simulink model "mrefrobotarm_modified_previous_y_previous_u_previous_ref_pert"  (R2018b)
settings: Solver=FixedStepAuto  StartTime=0.0  StopTime=10  RelTol=1e-3  AbsTol=1e-6
undefined symbols (not defined in the file or in its folder): cc, options
libraries: neural x714, simulink x1
(part 18 of 26)

== system mrefrobotarm_modified_previous_y_previous_u_previous_ref_pert/sd=0.01/Layer 3/Delays 1 ==
  "p{3}" : Inport  PortDimensions=30
      mask Display: e = 0.06;c1 = [120 230 180]/255;c2 = ([120 230 180]+0)/(256+128);c3 = ([120 230 180]+128)/(256+128);patch([0 1 1 0],[0 0 1 1],c1);patch([0 1 1 1-e 1-e 0+e],[0 0 1 1-e 0+e 0+e],c2);patch([0 0 1 1-e 0+e 0+e],[0 1 1 1-e 1-e 0+e],c3);plot([0 1 1 0 0],[0 0 1 1 0]);
  mux : Mux  Inputs=1
      mask Display: e = 0.06;c1 = [120 150 230]/255;c2 = ([120 150 230]+0)/383;c3 = ([120 150 230]+128)/383;patch([0 1 1 0],[0 0 1 1],c1);patch([0 1 1 1-e 1-e 0+e],[0 0 1 1-e 0+e 0+e],c2);patch([0 0 1 1-e 0+e 0+e],[0 1 1 1-e 1-e 0+e],c3);plot([0 1 1 0 0],[0 0 1 1 0]);disp('Mux')
  "pd{3,2}" : Outport
      mask Display: e = 0.06;c1 = [120 230 180]/255;c2 = ([120 230 180]+0)/(256+128);c3 = ([120 230 180]+128)/(256+128);patch([0 1 1 0],[0 0 1 1],c1);patch([0 1 1 1-e 1-e 0+e],[0 0 1 1-e 0+e 0+e],c2);patch([0 0 1 1-e 0+e 0+e],[0 1 1 1-e 1-e 0+e],c3);plot([0 1 1 0 0],[0 0 1 1 0]);
  wires:
  "p{3}"/1 -> mux/1
  mux/1 -> "pd{3,2}"/1

== system mrefrobotarm_modified_previous_y_previous_u_previous_ref_pert/sd=0.01/Layer 3/LW{3,2} ==
  "ad{3,2}" : Inport  PortDimensions=30
      mask Display: e = 0.06;c1 = [120 230 180]/255;c2 = ([120 230 180]+0)/(256+128);c3 = ([120 230 180]+128)/(256+128);patch([0 1 1 0],[0 0 1 1],c1);patch([0 1 1 1-e 1-e 0+e],[0 0 1 1-e 0+e 0+e],c2);patch([0 0 1 1-e 0+e 0+e],[0 1 1 1-e 1-e 0+e],c3);plot([0 1 1 0 0],[0 0 1 1 0]);
  "IW{3,2}(1,:)'" : Constant  Value=[-0.64661080882801724722952485535643063485622406005859375;0.122506844708924533815519453128217719495296478271484375;-0.1598857817103115086521114562856382690370082855224609375;0.763629292094280653913074274896644055843353271484375;0.64783885944440944282263217246509157121181488037109375;-0.36352935298451505286010387862916104495525360107421875;-0.43128711595355684327302014935412444174289703369140625;-0.5895897301103618648454585127183236181735992431640625;-0.08369026570109527884966382771381177008152008056640625;-0.1004753957202015046679122178829857148230075836181640625;-0.32808404490869491620941289511392824351787567138671875;0.32998136189090920833422160285408608615398406982421875;-0.4486208899527432958365125159616582095623016357421875;0.0261813632498970362549872703539222129620611667633056640625;0.282027752833665268372698164967005141079425811767578125;-0.018494292466418822684648404219842632301151752471923828125;-0.1400613205037356812088233937174663878977298736572265625;0.017723947989941535308133779835770837962627410888671875;-0.012245723361617721902661060084938071668148040771484375;0.10735791327470788070197471597566618584096431732177734375;-0.12221158004853945044931862184967030771076679229736328125;-0.101564950316621105397274504866800270974636077880859375;0.022351703842111880771170717707718722522258758544921875;-0.075846949807921060227045018109492957592010498046875;0.09973817654474255445240515882687759585678577423095703125;0.1126567720389630988808704614712041802704334259033203125;0.023371450347008236592127872199853300116956233978271484375;0.297336107042620145790579044842161238193511962890625;-0.319404206955927250088933533334056846797466278076171875;-0.48364044976087694482913548199576325714588165283203125]
      mask Display: e = 0.06;c1 = [120 150 230]/255;c2 = ([120 150 230]+0)/383;c3 = ([120 150 230]+128)/383;patch([0 1 1 0],[0 0 1 1],c1);patch([0 1 1 1-e 1-e 0+e],[0 0 1 1-e 0+e 0+e],c2);patch([0 0 1 1-e 0+e 0+e],[0 1 1 1-e 1-e 0+e],c3);plot([0 1 1 0 0],[0 0 1 1 0]);disp('weights');
  Mux : Mux  Inputs=1
      mask Display: e = 0.06;c1 = [120 150 230]/255;c2 = ([120 150 230]+0)/383;c3 = ([120 150 230]+128)/383;patch([0 1 1 0],[0 0 1 1],c1);patch([0 1 1 1-e 1-e 0+e],[0 0 1 1-e 0+e 0+e],c2);patch([0 0 1 1-e 0+e 0+e],[0 1 1 1-e 1-e 0+e],c3);plot([0 1 1 0 0],[0 0 1 1 0]);disp('Mux');
  dotprod1 : neural/Weight Functions/dotprod
  "lz{3,2}" : Outport
      mask Display: e = 0.06;c1 = [120 230 180]/255;c2 = ([120 230 180]+0)/(256+128);c3 = ([120 230 180]+128)/(256+128);patch([0 1 1 0],[0 0 1 1],c1);patch([0 1 1 1-e 1-e 0+e],[0 0 1 1-e 0+e 0+e],c2);patch([0 0 1 1-e 0+e 0+e],[0 1 1 1-e 1-e 0+e],c3);plot([0 1 1 0 0],[0 0 1 1 0]);
  wires:
  "IW{3,2}(1,:)'"/1 -> dotprod1/1
  "ad{3,2}"/1 -> dotprod1/2
  dotprod1/1 -> Mux/1
  Mux/1 -> "lz{3,2}"/1

== system mrefrobotarm_modified_previous_y_previous_u_previous_ref_pert/sd=0.1/Layer 1/Delays 1 ==
  "p{1}" : Inport  PortDimensions=10
      mask Display: e = 0.06;c1 = [120 230 180]/255;c2 = ([120 230 180]+0)/(256+128);c3 = ([120 230 180]+128)/(256+128);patch([0 1 1 0],[0 0 1 1],c1);patch([0 1 1 1-e 1-e 0+e],[0 0 1 1-e 0+e 0+e],c2);patch([0 0 1 1-e 0+e 0+e],[0 1 1 1-e 1-e 0+e],c3);plot([0 1 1 0 0],[0 0 1 1 0]);
  mux : Mux  Inputs=1
      mask Display: e = 0.06;c1 = [120 150 230]/255;c2 = ([120 150 230]+0)/383;c3 = ([120 150 230]+128)/383;patch([0 1 1 0],[0 0 1 1],c1);patch([0 1 1 1-e 1-e 0+e],[0 0 1 1-e 0+e 0+e],c2);patch([0 0 1 1-e 0+e 0+e],[0 1 1 1-e 1-e 0+e],c3);plot([0 1 1 0 0],[0 0 1 1 0]);disp('Mux')
  "pd{1,1}" : Outport
      mask Display: e = 0.06;c1 = [120 230 180]/255;c2 = ([120 230 180]+0)/(256+128);c3 = ([120 230 180]+128)/(256+128);patch([0 1 1 0],[0 0 1 1],c1);patch([0 1 1 1-e 1-e 0+e],[0 0 1 1-e 0+e 0+e],c2);patch([0 0 1 1-e 0+e 0+e],[0 1 1 1-e 1-e 0+e],c3);plot([0 1 1 0 0],[0 0 1 1 0]);
  wires:
  "p{1}"/1 -> mux/1
  mux/1 -> "pd{1,1}"/1

== system mrefrobotarm_modified_previous_y_previous_u_previous_ref_pert/sd=0.1/Layer 1/IW{1,1} ==
  "pd{1,1}" : Inport  PortDimensions=10
      mask Display: e = 0.06;c1 = [120 230 180]/255;c2 = ([120 230 180]+0)/(256+128);c3 = ([120 230 180]+128)/(256+128);patch([0 1 1 0],[0 0 1 1],c1);patch([0 1 1 1-e 1-e 0+e],[0 0 1 1-e 0+e 0+e],c2);patch([0 0 1 1-e 0+e 0+e],[0 1 1 1-e 1-e 0+e],c3);plot([0 1 1 0 0],[0 0 1 1 0]);
  "IW{1,1}(1,:)'" : Constant  Value=[5.6909541676817223532225398230366408824920654296875;-4.44478226511212515248416821123100817203521728515625;-0.69604359596750364769235375206335447728633880615234375;1.619034904975128252857530242181383073329925537109375;1.860125505340791907116226866492070257663726806640625;0.82729353143531325631698791767121292650699615478515625;-0.76269359990041951657957497445750050246715545654296875;-0.227256476361503645389205985338776372373104095458984375;0.461910119411805875078158578617149032652378082275390625;0.795152404857870198640057424199767410755157470703125]
      mask Display: e = 0.06;c1 = [120 150 230]/255;c2 = ([120 150 230]+0)/383;c3 = ([120 150 230]+128)/383;patch([0 1 1 0],[0 0 1 1],c1);patch([0 1 1 1-e 1-e 0+e],[0 0 1 1-e 0+e 0+e],c2);patch([0 0 1 1-e 0+e 0+e],[0 1 1 1-e 1-e 0+e],c3);plot([0 1 1 0 0],[0 0 1 1 0]);disp('Weights');
  "IW{1,1}(10,:)'" : Constant  Value=[3.77468306817619936310848061111755669116973876953125;-3.808687190450835924337980031850747764110565185546875;0.51746378608962484424438343921792693436145782470703125;-0.55078587150574531694502411482972092926502227783203125;-2.32173055805795680583969442523084580898284912109375;1.0626571361019880868070686119608581066131591796875;-0.23445984031463940056028150138445198535919189453125;-0.6493437208006149763406256170128472149372100830078125;1.4139047823904089540292261517606675624847412109375;0.617736660902912237958162222639657557010650634765625]
      mask Display: e = 0.06;c1 = [120 150 230]/255;c2 = ([120 150 230]+0)/383;c3 = ([120 150 230]+128)/383;patch([0 1 1 0],[0 0 1 1],c1);patch([0 1 1 1-e 1-e 0+e],[0 0 1 1-e 0+e 0+e],c2);patch([0 0 1 1-e 0+e 0+e],[0 1 1 1-e 1-e 0+e],c3);plot([0 1 1 0 0],[0 0 1 1 0]);disp('Weights');
  "IW{1,1}(11,:)'" : Constant  Value=[-0.1323443689410443990794874480343423783779144287109375;2.220754767172888222148685599677264690399169921875;11.4959613192428538042122454498894512653350830078125;-14.297590523719986066453202511183917522430419921875;-0.29115584099639824078309402466402389109134674072265625;3.022911440482079825642358628101646900177001953125;-0.112180835536244638550584795666509307920932769775390625;-0.981954934883976005011163579183630645275115966796875;0.10516967591617638888568109223342617042362689971923828125;1.8918544992947972094299302625586278736591339111328125]
      mask Display: e = 0.06;c1 = [120 150 230]/255;c2 = ([120 150 230]+0)/383;c3 = ([120 150 230]+128)/383;patch([0 1 1 0],[0 0 1 1],c1);patch([0 1 1 1-e 1-e 0+e],[0 0 1 1-e 0+e 0+e],c2);patch([0 0 1 1-e 0+e 0+e],[0 1 1 1-e 1-e 0+e],c3);plot([0 1 1 0 0],[0 0 1 1 0]);disp('Weights');
  "IW{1,1}(12,:)'" : Constant  Value=[0.72754685821430609138360523502342402935028076171875;-0.6570666137841676412989500022376887500286102294921875;-0.307371304859638871942451032737153582274913787841796875;-0.058820122292903016802956273068048176355659961700439453125;0.161741526428527071512775137307471595704555511474609375;-0.05792305025135065232877451535387081094086170196533203125;1.180419195584523794906317561981268227100372314453125;-0.51747520174959993344288022854016162455081939697265625;0.305574366681974851633896150815417058765888214111328125;0.2273021954544744149817603329211124219000339508056640625]
      mask Display: e = 0.06;c1 = [120 150 230]/255;c2 = ([120 150 230]+0)/383;c3 = ([120 150 230]+128)/383;patch([0 1 1 0],[0 0 1 1],c1);patch([0 1 1 1-e 1-e 0+e],[0 0 1 1-e 0+e 0+e],c2);patch([0 0 1 1-e 0+e 0+e],[0 1 1 1-e 1-e 0+e],c3);plot([0 1 1 0 0],[0 0 1 1 0]);disp('Weights');
  "IW{1,1}(13,:)'" : Constant  Value=[0.92475187713074102902055528829805552959442138671875;-0.7246700213142720503611826643464155495166778564453125;-0.54231701267272092170657060705707408487796783447265625;-0.74731381930544571456920266427914611995220184326171875;-0.37753760663786517515205787276499904692173004150390625;0.69288465345196315059439484684844501316547393798828125;-0.6787969769950346066167412573122419416904449462890625;1.4879723311172383670708541103522293269634246826171875;1.0728866219769777057280180088127963244915008544921875;-0.0257443446317741110596077902528122649528086185455322265625]
      mask Display: e = 0.06;c1 = [120 150 230]/255;c2 = ([120 150 230]+0)/383;c3 = ([120 150 230]+128)/383;patch([0 1 1 0],[0 0 1 1],c1);patch([0 1 1 1-e 1-e 0+e],[0 0 1 1-e 0+e 0+e],c2);patch([0 0 1 1-e 0+e 0+e],[0 1 1 1-e 1-e 0+e],c3);plot([0 1 1 0 0],[0 0 1 1 0]);disp('Weights');
  "IW{1,1}(14,:)'" : Constant  Value=[-0.39658704580621850777077952443505637347698211669921875;-2.570658577061915917028045441838912665843963623046875;2.097471663743316838690589065663516521453857421875;-0.182743645563124779140906639440800063312053680419921875;3.173197263880643159694727728492580354213714599609375;-2.566203225034959789496724624768830835819244384765625;0.28465571871831463202084933072910644114017486572265625;0.53816262288512628497727519061299972236156463623046875;1.148349370577057104725327008054591715335845947265625;-0.77361570994371497977937224277411587536334991455078125]
      mask Display: e = 0.06;c1 = [120 150 230]/255;c2 = ([120 150 230]+0)/383;c3 = ([120 150 230]+128)/383;patch([0 1 1 0],[0 0 1 1],c1);patch([0 1 1 1-e 1-e 0+e],[0 0 1 1-e 0+e 0+e],c2);patch([0 0 1 1-e 0+e 0+e],[0 1 1 1-e 1-e 0+e],c3);plot([0 1 1 0 0],[0 0 1 1 0]);disp('Weights');
  "IW{1,1}(15,:)'" : Constant  Value=[-1.233071996055086660959432265372015535831451416015625;3.729934935631209924622453399933874607086181640625;-0.69194072859403676911682623540400527417659759521484375;-0.06934859583439123564829742463189177215099334716796875;-1.3472043188516165113099987138411961495876312255859375;0.088223980720888273143742708271020092070102691650390625;-0.7180079381626434109620049639488570392131805419921875;-0.050715270149810497135600684259770787321031093597412109375;-0.79841827776868690147438201165641658008098602294921875;0.6403567898287889637032321843435056507587432861328125]
      mask Display: e = 0.06;c1 = [120 150 230]/255;c2 = ([120 150 230]+0)/383;c3 = ([120 150 230]+128)/383;patch([0 1 1 0],[0 0 1 1],c1);patch([0 1 1 1-e 1-e 0+e],[0 0 1 1-e 0+e 0+e],c2);patch([0 0 1 1-e 0+e 0+e],[0 1 1 1-e 1-e 0+e],c3);plot([0 1 1 0 0],[0 0 1 1 0]);disp('Weights');
  "IW{1,1}(16,:)'" : Constant  Value=[-0.4501147463957007044399460937711410224437713623046875;-0.4634484641641158919611598321353085339069366455078125;-1.074232972538778252413749214611016213893890380859375;2.414632291410705011713844214682467281818389892578125;1.5871822908788753014874828295432962477207183837890625;-0.936050277862158441877227232907898724079132080078125;-0.301929298988273753234778951082262210547924041748046875;0.2105845785872021147522303863297565840184688568115234375;-0.389900971878246072055418380841729231178760528564453125;-0.34803444346408973775197637223755009472370147705078125]
      mask Display: e = 0.06;c1 = [120 150 230]/255;c2 = ([120 150 230]+0)/383;c3 = ([120 150 230]+128)/383;patch([0 1 1 0],[0 0 1 1],c1);patch([0 1 1 1-e 1-e 0+e],[0 0 1 1-e 0+e 0+e],c2);patch([0 0 1 1-e 0+e 0+e],[0 1 1 1-e 1-e 0+e],c3);plot([0 1 1 0 0],[0 0 1 1 0]);disp('Weights');
  "IW{1,1}(17,:)'" : Constant  Value=[-0.99686635965547853999169092276133596897125244140625;-4.42672798675833245596322740311734378337860107421875;0.52979427551061120116315805717022158205509185791015625;6.21254233611867245912208090885542333126068115234375;0.5363341023376178018366999822319485247135162353515625;-1.0699517545959584818859866572893224656581878662109375;2.39944942593691745713613272528164088726043701171875;0.260939315381722158893040841576294042170047760009765625;0.2099266373906171490038019555868231691420078277587890625;-0.994914330157364634743544229422695934772491455078125]
      mask Display: e = 0.06;c1 = [120 150 230]/255;c2 = ([120 150 230]+0)/383;c3 = ([120 150 230]+128)/383;patch([0 1 1 0],[0 0 1 1],c1);patch([0 1 1 1-e 1-e 0+e],[0 0 1 1-e 0+e 0+e],c2);patch([0 0 1 1-e 0+e 0+e],[0 1 1 1-e 1-e 0+e],c3);plot([0 1 1 0 0],[0 0 1 1 0]);disp('Weights');
  "IW{1,1}(18,:)'" : Constant  Value=[-0.821393751051058274015304050408303737640380859375;-0.01417692834606891494342306714315782301127910614013671875;2.038276852058502175424337110598571598529815673828125;-2.792063261322187628366009448654949665069580078125;0.2963152941576634447073956835083663463592529296875;1.2640438926848338585529063493595458567142486572265625;-0.435348179999016704488923323879134841263294219970703125;-0.73195572965866928516476264121592976152896881103515625;0.452296877126517726797061413890332914888858795166015625;0.4165847639021185155883131301379762589931488037109375]
      mask Display: e = 0.06;c1 = [120 150 230]/255;c2 = ([120 150 230]+0)/383;c3 = ([120 150 230]+128)/383;patch([0 1 1 0],[0 0 1 1],c1);patch([0 1 1 1-e 1-e 0+e],[0 0 1 1-e 0+e 0+e],c2);patch([0 0 1 1-e 0+e 0+e],[0 1 1 1-e 1-e 0+e],c3);plot([0 1 1 0 0],[0 0 1 1 0]);disp('Weights');
  "IW{1,1}(19,:)'" : Constant  Value=[-0.021101967185585483732790379463040153495967388153076171875;1.04526769321619639185882988385856151580810546875;1.5178135598712625409234533435665071010589599609375;-3.477264311782526373661994512076489627361297607421875;-0.65282281292846311426814054357237182557582855224609375;0.53320969745519108951015141428797505795955657958984375;-0.37582875730548692683186118301819078624248504638671875;-0.45838305167290815944625137490220367908477783203125;-0.74592449376494152080141475380514748394489288330078125;0.83188799160172621771636158882756717503070831298828125]
      mask Display: e = 0.06;c1 = [120 150 230]/255;c2 = ([120 150 230]+0)/383;c3 = ([120 150 230]+128)/383;patch([0 1 1 0],[0 0 1 1],c1);patch([0 1 1 1-e 1-e 0+e],[0 0 1 1-e 0+e 0+e],c2);patch([0 0 1 1-e 0+e 0+e],[0 1 1 1-e 1-e 0+e],c3);plot([0 1 1 0 0],[0 0 1 1 0]);disp('Weights');
  "IW{1,1}(2,:)'" : Constant  Value=[4.62277869178698352925493963994085788726806640625;-5.92539205904510435374277221853844821453094482421875;-5.55160319243273203682065286557190120220184326171875;6.302029269116832921326931682415306568145751953125;-2.388380381000120511458817418315447866916656494140625;2.719370242134512505316479291650466620922088623046875;1.95707593454640260688393027521669864654541015625;1.8905825205932362820249181822873651981353759765625;0.8757237097918684209929551798268221318721771240234375;-0.5701625650547226253905819248757325112819671630859375]
      mask Display: e = 0.06;c1 = [120 150 230]/255;c2 = ([120 150 230]+0)/383;c3 = ([120 150 230]+128)/383;patch([0 1 1 0],[0 0 1 1],c1);patch([0 1 1 1-e 1-e 0+e],[0 0 1 1-e 0+e 0+e],c2);patch([0 0 1 1-e 0+e 0+e],[0 1 1 1-e 1-e 0+e],c3);plot([0 1 1 0 0],[0 0 1 1 0]);disp('Weights');
  "IW{1,1}(20,:)'" : Constant  Value=[0.62919967447007685290571998848463408648967742919921875;0.63822100806571480102746818374725989997386932373046875;-2.558216234778203812538777128793299198150634765625;3.824630195820196920664102435694076120853424072265625;-1.3901016767274487762051649042405188083648681640625;-1.4697718575967773091406343155540525913238525390625;0.320656284353787179863815026692464016377925872802734375;0.03903647293257066219762663195069762878119945526123046875;-0.8694351181026103159155127286794595420360565185546875;-0.1668543775041878285403385007157339714467525482177734375]
      mask Display: e = 0.06;c1 = [120 150 230]/255;c2 = ([120 150 230]+0)/383;c3 = ([120 150 230]+128)/383;patch([0 1 1 0],[0 0 1 1],c1);patch([0 1 1 1-e 1-e 0+e],[0 0 1 1-e 0+e 0+e],c2);patch([0 0 1 1-e 0+e 0+e],[0 1 1 1-e 1-e 0+e],c3);plot([0 1 1 0 0],[0 0 1 1 0]);disp('Weights');
  "IW{1,1}(21,:)'" : Constant  Value=[-3.194363280613027544774240595870651304721832275390625;1.5297503007089605642221386005985550582408905029296875;-3.335353197396081714742877011303789913654327392578125;2.755968737305007021376468401285819709300994873046875;-1.1818578966401160901256162105710245668888092041015625;-0.07705839442231239566627465364945237524807453155517578125;-0.382468145323676844693494558669044636189937591552734375;-0.2534211222472129154681397267268039286136627197265625;-0.036089917237800604732367304450235678814351558685302734375;-1.125935256119358740534153184853494167327880859375]
      mask Display: e = 0.06;c1 = [120 150 230]/255;c2 = ([120 150 230]+0)/383;c3 = ([120 150 230]+128)/383;patch([0 1 1 0],[0 0 1 1],c1);patch([0 1 1 1-e 1-e 0+e],[0 0 1 1-e 0+e 0+e],c2);patch([0 0 1 1-e 0+e 0+e],[0 1 1 1-e 1-e 0+e],c3);plot([0 1 1 0 0],[0 0 1 1 0]);disp('Weights');
  "IW{1,1}(22,:)'" : Constant  Value=[-0.3879768225013970894821113688522018492221832275390625;0.65287118396852561463816755349398590624332427978515625;2.092411199976454749815957256942056119441986083984375;0.266824732827123434208971275438671000301837921142578125;0.83935601495915135306091769962222315371036529541015625;-0.999583256938282094239411890157498419284820556640625;1.6268816212547194677284778663306497037410736083984375;-2.15132497060458494075874114059843122959136962890625;-1.0817300961504832113035945440060459077358245849609375;-0.1348446343211972264786169262151815928518772125244140625]
      mask Display: e = 0.06;c1 = [120 150 230]/255;c2 = ([120 150 230]+0)/383;c3 = ([120 150 230]+128)/383;patch([0 1 1 0],[0 0 1 1],c1);patch([0 1 1 1-e 1-e 0+e],[0 0 1 1-e 0+e 0+e],c2);patch([0 0 1 1-e 0+e 0+e],[0 1 1 1-e 1-e 0+e],c3);plot([0 1 1 0 0],[0 0 1 1 0]);disp('Weights');
  "IW{1,1}(23,:)'" : Constant  Value=[0.93645641909832699756321972017758525907993316650390625;-1.1635179598223779340315786612336523830890655517578125;-1.2315261915118025370929899509064853191375732421875;0.20667802205517993296979284423287026584148406982421875;-5.3037751841913571837494600913487374782562255859375;1.1584284966934494942591982180601917207241058349609375;-0.9775638083026090274785246947431005537509918212890625;2.85546522193933061117832039599306881427764892578125;-0.9535912297005648685654932705801911652088165283203125;-0.498925158764337961514456765144132077693939208984375]
      mask Display: e = 0.06;c1 = [120 150 230]/255;c2 = ([120 150 230]+0)/383;c3 = ([120 150 230]+128)/383;patch([0 1 1 0],[0 0 1 1],c1);patch([0 1 1 1-e 1-e 0+e],[0 0 1 1-e 0+e 0+e],c2);patch([0 0 1 1-e 0+e 0+e],[0 1 1 1-e 1-e 0+e],c3);plot([0 1 1 0 0],[0 0 1 1 0]);disp('Weights');
  "IW{1,1}(24,:)'" : Constant  Value=[2.70451824343148228280142575385980308055877685546875;-2.227798650416434877996607610839419066905975341796875;-0.3298847619577129908208235065103508532047271728515625;-0.89481065329824038823147702714777551591396331787109375;-0.52466488972875569007925378173240460455417633056640625;1.710805285647084783562377197085879743099212646484375;1.031854828812333924048516564653255045413970947265625;1.1086282305300176886930785258300602436065673828125;-0.14372450255704538601975173151004128158092498779296875;0.02890495460854762554969710208752076141536235809326171875]
      mask Display: e = 0.06;c1 = [120 150 230]/255;c2 = ([120 150 230]+0)/383;c3 = ([120 150 230]+128)/383;patch([0 1 1 0],[0 0 1 1],c1);patch([0 1 1 1-e 1-e 0+e],[0 0 1 1-e 0+e 0+e],c2);patch([0 0 1 1-e 0+e 0+e],[0 1 1 1-e 1-e 0+e],c3);plot([0 1 1 0 0],[0 0 1 1 0]);disp('Weights');
  "IW{1,1}(25,:)'" : Constant  Value=[-2.895961697780943477908977001789025962352752685546875;1.0162975636695488201866055533173494040966033935546875;-0.318323957164946824693885218948707915842533111572265625;-0.95893038462431012813880215617245994508266448974609375;-2.53127470879748894816430038190446794033050537109375;2.727790700757982023105796542949974536895751953125;-0.1428332212615507634811962134335772134363651275634765625;-1.7529138492328291132338335955864749848842620849609375;-0.67137994434078029915013985373661853373050689697265625;0.136353975516636138909376541050733067095279693603515625]
      mask Display: e = 0.06;c1 = [120 150 230]/255;c2 = ([120 150 230]+0)/383;c3 = ([120 150 230]+128)/383;patch([0 1 1 0],[0 0 1 1],c1);patch([0 1 1 1-e 1-e 0+e],[0 0 1 1-e 0+e 0+e],c2);patch([0 0 1 1-e 0+e 0+e],[0 1 1 1-e 1-e 0+e],c3);plot([0 1 1 0 0],[0 0 1 1 0]);disp('Weights');
  "IW{1,1}(26,:)'" : Constant  Value=[7.112248552032273352097035967744886875152587890625;-4.33679686775016559607820454402826726436614990234375;-0.93254371888148834823795141346636228263378143310546875;1.2568127272896345569819231968722306191921234130859375;-0.56591244280561758817071904559270478785037994384765625;0.495033476999858168543511283132829703390598297119140625;2.072134510876653568089977852650918066501617431640625;0.58980333857500200078760599353699944913387298583984375;1.47600055081548564572813120321370661258697509765625;3.262771438757822384246765068382956087589263916015625]
      mask Display: e = 0.06;c1 = [120 150 230]/255;c2 = ([120 150 230]+0)/383;c3 = ([120 150 230]+128)/383;patch([0 1 1 0],[0 0 1 1],c1);patch([0 1 1 1-e 1-e 0+e],[0 0 1 1-e 0+e 0+e],c2);patch([0 0 1 1-e 0+e 0+e],[0 1 1 1-e 1-e 0+e],c3);plot([0 1 1 0 0],[0 0 1 1 0]);disp('Weights');
  "IW{1,1}(27,:)'" : Constant  Value=[-0.1809479253412995258809559118162724189460277557373046875;1.3329712715830945857220513062202371656894683837890625;-0.727829017689943125191120998351834714412689208984375;-0.0865326110248336444197292394164833240211009979248046875;-1.585325797544271164696283449302427470684051513671875;0.822739914311575670780030122841708362102508544921875;0.05187354196452260979288695352806826122105121612548828125;0.2353588101939095567072257608742802403867244720458984375;-0.83603218726290517981425409743678756058216094970703125;-0.0278576384392767717468331056807073764503002166748046875]
      mask Display: e = 0.06;c1 = [120 150 230]/255;c2 = ([120 150 230]+0)/383;c3 = ([120 150 230]+128)/383;patch([0 1 1 0],[0 0 1 1],c1);patch([0 1 1 1-e 1-e 0+e],[0 0 1 1-e 0+e 0+e],c2);patch([0 0 1 1-e 0+e 0+e],[0 1 1 1-e 1-e 0+e],c3);plot([0 1 1 0 0],[0 0 1 1 0]);disp('Weights');
  "IW{1,1}(28,:)'" : Constant  Value=[-0.25988610528345679195894035728997550904750823974609375;-0.783303336113111203786729674902744591236114501953125;1.6978153364625587773417692005750723183155059814453125;0.1615124990326344545099601646143128164112567901611328125;-0.25572632437584019715615113454987294971942901611328125;-0.1379086778636360588468079413360101170837879180908203125;0.081340999105558864368248350729118101298809051513671875;0.7546077921921525710757805427419953048229217529296875;1.78061266540529938851022961898706853389739990234375;1.2173461383866592822045049615553580224514007568359375]
      mask Display: e = 0.06;c1 = [120 150 230]/255;c2 = ([120 150 230]+0)/383;c3 = ([120 150 230]+128)/383;patch([0 1 1 0],[0 0 1 1],c1);patch([0 1 1 1-e 1-e 0+e],[0 0 1 1-e 0+e 0+e],c2);patch([0 0 1 1-e 0+e 0+e],[0 1 1 1-e 1-e 0+e],c3);plot([0 1 1 0 0],[0 0 1 1 0]);disp('Weights');
  "IW{1,1}(29,:)'" : Constant  Value=[3.838440868156633545282829800271429121494293212890625;6.37405974419134135899867033003829419612884521484375;-14.4249463973180684916997051914222538471221923828125;-4.5941903300428332812543885665945708751678466796875;0.27248272559942687820466744597069919109344482421875;1.7863221628485443925882236726465635001659393310546875;0.0018237333289003072878120548239166964776813983917236328125;0.84334663848897972737717054769746027886867523193359375;-0.61127312655363097437799524414003826677799224853515625;1.295663177400013577056370195350609719753265380859375]
      mask Display: e = 0.06;c1 = [120 150 230]/255;c2 = ([120 150 230]+0)/383;c3 = ([120 150 230]+128)/383;patch([0 1 1 0],[0 0 1 1],c1);patch([0 1 1 1-e 1-e 0+e],[0 0 1 1-e 0+e 0+e],c2);patch([0 0 1 1-e 0+e 0+e],[0 1 1 1-e 1-e 0+e],c3);plot([0 1 1 0 0],[0 0 1 1 0]);disp('Weights');
  "IW{1,1}(3,:)'" : Constant  Value=[-0.95335229790588638110193642205558717250823974609375;0.8135858620981608613220714687486179172992706298828125;1.0561197407740365861172904260456562042236328125;-0.353428658818821073150928668837877921760082244873046875;-1.152329760314444673241496275295503437519073486328125;0.881537554780707832691177827655337750911712646484375;-0.040331396959935615631476224507423467002809047698974609375;0.388676217778073762598722851180355064570903778076171875;0.46716977742257526085012386829475872218608856201171875;0.42630078372956548005134891354828141629695892333984375]
      mask Display: e = 0.06;c1 = [120 150 230]/255;c2 = ([120 150 230]+0)/383;c3 = ([120 150 230]+128)/383;patch([0 1 1 0],[0 0 1 1],c1);patch([0 1 1 1-e 1-e 0+e],[0 0 1 1-e 0+e 0+e],c2);patch([0 0 1 1-e 0+e 0+e],[0 1 1 1-e 1-e 0+e],c3);plot([0 1 1 0 0],[0 0 1 1 0]);disp('Weights');
  "IW{1,1}(30,:)'" : Constant  Value=[-1.623668586828416859901835778146050870418548583984375;0.278185668845817024585898025179631076753139495849609375;2.010439965225419900463066369411535561084747314453125;0.9017129401025527624113919955561868846416473388671875;-0.7755659660602718386002152328728698194026947021484375;-1.548090584963351279412790972855873405933380126953125;-2.14538957718599920809765535523183643817901611328125;-0.505301029911102705938219514791853725910186767578125;2.515454711856583980278401213581673800945281982421875;1.0292747210291126602754729901789687573909759521484375]
      mask Display: e = 0.06;c1 = [120 150 230]/255;c2 = ([120 150 230]+0)/383;c3 = ([120 150 230]+128)/383;patch([0 1 1 0],[0 0 1 1],c1);patch([0 1 1 1-e 1-e 0+e],[0 0 1 1-e 0+e 0+e],c2);patch([0 0 1 1-e 0+e 0+e],[0 1 1 1-e 1-e 0+e],c3);plot([0 1 1 0 0],[0 0 1 1 0]);disp('Weights');
  "IW{1,1}(4,:)'" : Constant  Value=[1.724590481369361771868398136575706303119659423828125;-1.1802329338394199620410063289455138146877288818359375;-3.228648492999071084597062508692033588886260986328125;1.8663066072214016255514934528036974370479583740234375;-0.24207628261569891225946093982202000916004180908203125;1.0791692509266415100910307955928146839141845703125;-1.8094766078651589591430592918186448514461517333984375;2.5199304877392716406347972224466502666473388671875;-0.1485285343659628887191814783363952301442623138427734375;1.310200383499971366063618916086852550506591796875]
      mask Display: e = 0.06;c1 = [120 150 230]/255;c2 = ([120 150 230]+0)/383;c3 = ([120 150 230]+128)/383;patch([0 1 1 0],[0 0 1 1],c1);patch([0 1 1 1-e 1-e 0+e],[0 0 1 1-e 0+e 0+e],c2);patch([0 0 1 1-e 0+e 0+e],[0 1 1 1-e 1-e 0+e],c3);plot([0 1 1 0 0],[0 0 1 1 0]);disp('Weights');
  "IW{1,1}(5,:)'" : Constant  Value=[0.07095244958430364790036293243247200734913349151611328125;-0.6585017123226279966985430291970260441303253173828125;0.350039503563764842208883010243880562484264373779296875;0.139066788886854697526729296441772021353244781494140625;0.789178234463720595925906309275887906551361083984375;-0.41575257001524923428092961330548860132694244384765625;-0.1127560859663192249779939402287709526717662811279296875;-0.185613729077827194213767825203831307590007781982421875;0.572655777628925388711422783671878278255462646484375;0.07108288206217704130462919920319109223783016204833984375]
      mask Display: e = 0.06;c1 = [120 150 230]/255;c2 = ([120 150 230]+0)/383;c3 = ([120 150 230]+128)/383;patch([0 1 1 0],[0 0 1 1],c1);patch([0 1 1 1-e 1-e 0+e],[0 0 1 1-e 0+e 0+e],c2);patch([0 0 1 1-e 0+e 0+e],[0 1 1 1-e 1-e 0+e],c3);plot([0 1 1 0 0],[0 0 1 1 0]);disp('Weights');
  "IW{1,1}(6,:)'" : Constant  Value=[-2.383575448051668654869672536733560264110565185546875;2.911302734219824994710279497667215764522552490234375;-0.333866900586164472297667771272244863212108612060546875;0.1902957702433549502796239494273322634398937225341796875;0.61826176421184175779899305780418217182159423828125;-0.305137527239768335807212906729546375572681427001953125;-0.58919389025756940814204654088825918734073638916015625;0.2495788997447347112856874673525453545153141021728515625;1.328162244689349957837976035079918801784515380859375;0.443461835124141057207225458114407956600189208984375]
      mask Display: e = 0.06;c1 = [120 150 230]/255;c2 = ([120 150 230]+0)/383;c3 = ([120 150 230]+128)/383;patch([0 1 1 0],[0 0 1 1],c1);patch([0 1 1 1-e 1-e 0+e],[0 0 1 1-e 0+e 0+e],c2);patch([0 0 1 1-e 0+e 0+e],[0 1 1 1-e 1-e 0+e],c3);plot([0 1 1 0 0],[0 0 1 1 0]);disp('Weights');
  "IW{1,1}(7,:)'" : Constant  Value=[0.370945242004492248266700471504009328782558441162109375;-0.89895476380015626460817657061852514743804931640625;0.85290707165510493137361436311039142310619354248046875;-0.08983671164446171975015431598876602947711944580078125;-0.7836981741913107146757511145551688969135284423828125;0.73082442816330839274741038025240413844585418701171875;0.005763866157285656155462305605396977625787258148193359375;-0.2735757805697185407467486584209837019443511962890625;-0.143162208450970329653983981188503094017505645751953125;0.35728592684730298145723281777463853359222412109375]
      mask Display: e = 0.06;c1 = [120 150 230]/255;c2 = ([120 150 230]+0)/383;c3 = ([120 150 230]+128)/383;patch([0 1 1 0],[0 0 1 1],c1);patch([0 1 1 1-e 1-e 0+e],[0 0 1 1-e 0+e 0+e],c2);patch([0 0 1 1-e 0+e 0+e],[0 1 1 1-e 1-e 0+e],c3);plot([0 1 1 0 0],[0 0 1 1 0]);disp('Weights');
  "IW{1,1}(8,:)'" : Constant  Value=[2.493414744591201159806814757757820188999176025390625;-1.1478004266133201571875588342663832008838653564453125;-1.5184808259941646735313725002924911677837371826171875;4.13179970627668158300593859166838228702545166015625;-2.86947679435950586679382467991672456264495849609375;-1.455006878714796503260231474996544420719146728515625;1.1892376296648994316029757101205177605152130126953125;-1.585663123861548395865384009084664285182952880859375;1.1973568861551127096021218676469288766384124755859375;-0.502886716778984332876234475406818091869354248046875]
      mask Display: e = 0.06;c1 = [120 150 230]/255;c2 = ([120 150 230]+0)/383;c3 = ([120 150 230]+128)/383;patch([0 1 1 0],[0 0 1 1],c1);patch([0 1 1 1-e 1-e 0+e],[0 0 1 1-e 0+e 0+e],c2);patch([0 0 1 1-e 0+e 0+e],[0 1 1 1-e 1-e 0+e],c3);plot([0 1 1 0 0],[0 0 1 1 0]);disp('Weights');
  "IW{1,1}(9,:)'" : Constant  Value=[-0.688891163973588849245288656675256788730621337890625;1.40543679990872849572269842610694468021392822265625;0.57698786730975826220202407057513482868671417236328125;-0.75128518614270711761804477646364830434322357177734375;-0.878513359396675408419241648516617715358734130859375;-0.75939164292714467219269636188982985913753509521484375;-1.2591782208006685461754159405245445668697357177734375;-0.4865913520035707318101003693300299346446990966796875;0.612347477969967801669781692908145487308502197265625;1.349737428105989511806228620116598904132843017578125]
      mask Display: e = 0.06;c1 = [120 150 230]/255;c2 = ([120 150 230]+0)/383;c3 = ([120 150 230]+128)/383;patch([0 1 1 0],[0 0 1 1],c1);patch([0 1 1 1-e 1-e 0+e],[0 0 1 1-e 0+e 0+e],c2);patch([0 0 1 1-e 0+e 0+e],[0 1 1 1-e 1-e 0+e],c3);plot([0 1 1 0 0],[0 0 1 1 0]);disp('Weights');
  Mux : Mux  Inputs=30
      mask Display: e = 0.06;c1 = [120 150 230]/255;c2 = ([120 150 230]+0)/383;c3 = ([120 150 230]+128)/383;patch([0 1 1 0],[0 0 1 1],c1);patch([0 1 1 1-e 1-e 0+e],[0 0 1 1-e 0+e 0+e],c2);patch([0 0 1 1-e 0+e 0+e],[0 1 1 1-e 1-e 0+e],c3);plot([0 1 1 0 0],[0 0 1 1 0]);disp('Mux');
  dotprod{1..30} (30 alike) : neural/Weight Functions/dotprod
  "iz{1,1}" : Outport
      mask Display: e = 0.06;c1 = [120 230 180]/255;c2 = ([120 230 180]+0)/(256+128);c3 = ([120 230 180]+128)/(256+128);patch([0 1 1 0],[0 0 1 1],c1);patch([0 1 1 1-e 1-e 0+e],[0 0 1 1-e 0+e 0+e],c2);patch([0 0 1 1-e 0+e 0+e],[0 1 1 1-e 1-e 0+e],c3);plot([0 1 1 0 0],[0 0 1 1 0]);
  wires:
  "IW{1,1}(1,:)'"/1 -> dotprod1/1
  "pd{1,1}"/1 -> dotprod1/2, dotprod2/2, dotprod3/2, dotprod4/2, dotprod5/2, dotprod6/2, dotprod7/2, dotprod8/2, dotprod9/2, dotprod10/2, dotprod11/2, dotprod12/2, dotprod13/2, dotprod14/2, dotprod15/2, dotprod16/2, dotprod17/2, dotprod18/2, dotprod19/2, dotprod20/2, dotprod21/2, dotprod22/2, dotprod23/2, dotprod24/2, dotprod25/2, dotprod26/2, dotprod27/2, dotprod28/2, dotprod29/2, dotprod30/2
  dotprod1/1 -> Mux/1
  "IW{1,1}(2,:)'"/1 -> dotprod2/1
  dotprod2/1 -> Mux/2
  "IW{1,1}(3,:)'"/1 -> dotprod3/1
  dotprod3/1 -> Mux/3
  "IW{1,1}(4,:)'"/1 -> dotprod4/1
  dotprod4/1 -> Mux/4
  "IW{1,1}(5,:)'"/1 -> dotprod5/1
  dotprod5/1 -> Mux/5
  "IW{1,1}(6,:)'"/1 -> dotprod6/1
  dotprod6/1 -> Mux/6
  "IW{1,1}(7,:)'"/1 -> dotprod7/1
  dotprod7/1 -> Mux/7
  "IW{1,1}(8,:)'"/1 -> dotprod8/1
  dotprod8/1 -> Mux/8
  "IW{1,1}(9,:)'"/1 -> dotprod9/1
  dotprod9/1 -> Mux/9
  "IW{1,1}(10,:)'"/1 -> dotprod10/1
  dotprod10/1 -> Mux/10
  "IW{1,1}(11,:)'"/1 -> dotprod11/1
  dotprod11/1 -> Mux/11
  "IW{1,1}(12,:)'"/1 -> dotprod12/1
  dotprod12/1 -> Mux/12
  "IW{1,1}(13,:)'"/1 -> dotprod13/1
  dotprod13/1 -> Mux/13
  "IW{1,1}(14,:)'"/1 -> dotprod14/1
  dotprod14/1 -> Mux/14
  "IW{1,1}(15,:)'"/1 -> dotprod15/1
  dotprod15/1 -> Mux/15
  "IW{1,1}(16,:)'"/1 -> dotprod16/1
  dotprod16/1 -> Mux/16
  "IW{1,1}(17,:)'"/1 -> dotprod17/1
  dotprod17/1 -> Mux/17
  "IW{1,1}(18,:)'"/1 -> dotprod18/1
  dotprod18/1 -> Mux/18
  "IW{1,1}(19,:)'"/1 -> dotprod19/1
  dotprod19/1 -> Mux/19
  "IW{1,1}(20,:)'"/1 -> dotprod20/1
  dotprod20/1 -> Mux/20
  "IW{1,1}(21,:)'"/1 -> dotprod21/1
  dotprod21/1 -> Mux/21
  "IW{1,1}(22,:)'"/1 -> dotprod22/1
  dotprod22/1 -> Mux/22
  "IW{1,1}(23,:)'"/1 -> dotprod23/1
  dotprod23/1 -> Mux/23
  "IW{1,1}(24,:)'"/1 -> dotprod24/1
  dotprod24/1 -> Mux/24
  "IW{1,1}(25,:)'"/1 -> dotprod25/1
  dotprod25/1 -> Mux/25
  "IW{1,1}(26,:)'"/1 -> dotprod26/1
  dotprod26/1 -> Mux/26
  "IW{1,1}(27,:)'"/1 -> dotprod27/1
  dotprod27/1 -> Mux/27
  "IW{1,1}(28,:)'"/1 -> dotprod28/1
  dotprod28/1 -> Mux/28
  "IW{1,1}(29,:)'"/1 -> dotprod29/1
  dotprod29/1 -> Mux/29
  "IW{1,1}(30,:)'"/1 -> dotprod30/1
  dotprod30/1 -> Mux/30
  Mux/1 -> "iz{1,1}"/1

== system mrefrobotarm_modified_previous_y_previous_u_previous_ref_pert/sd=0.1/Layer 2/Delays 1 ==
  "p{2}" : Inport  PortDimensions=30
      mask Display: e = 0.06;c1 = [120 230 180]/255;c2 = ([120 230 180]+0)/(256+128);c3 = ([120 230 180]+128)/(256+128);patch([0 1 1 0],[0 0 1 1],c1);patch([0 1 1 1-e 1-e 0+e],[0 0 1 1-e 0+e 0+e],c2);patch([0 0 1 1-e 0+e 0+e],[0 1 1 1-e 1-e 0+e],c3);plot([0 1 1 0 0],[0 0 1 1 0]);
  mux : Mux  Inputs=1
      mask Display: e = 0.06;c1 = [120 150 230]/255;c2 = ([120 150 230]+0)/383;c3 = ([120 150 230]+128)/383;patch([0 1 1 0],[0 0 1 1],c1);patch([0 1 1 1-e 1-e 0+e],[0 0 1 1-e 0+e 0+e],c2);patch([0 0 1 1-e 0+e 0+e],[0 1 1 1-e 1-e 0+e],c3);plot([0 1 1 0 0],[0 0 1 1 0]);disp('Mux')
  "pd{2,1}" : Outport
      mask Display: e = 0.06;c1 = [120 230 180]/255;c2 = ([120 230 180]+0)/(256+128);c3 = ([120 230 180]+128)/(256+128);patch([0 1 1 0],[0 0 1 1],c1);patch([0 1 1 1-e 1-e 0+e],[0 0 1 1-e 0+e 0+e],c2);patch([0 0 1 1-e 0+e 0+e],[0 1 1 1-e 1-e 0+e],c3);plot([0 1 1 0 0],[0 0 1 1 0]);
  wires:
  "p{2}"/1 -> mux/1
  mux/1 -> "pd{2,1}"/1
